simulink model "Helicopter_Model"  (R2025a)
settings: Solver=VariableStepAuto  StartTime=0.0  StopTime=10.0  RelTol=1e-3
settings Model: Creator=Admin  LastModifiedBy=Admin

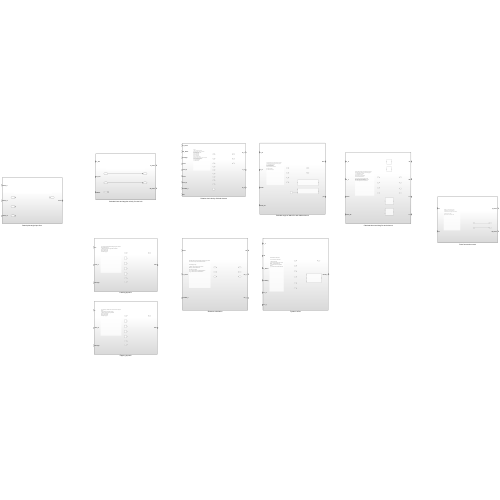
[thumbnail: Simulink's stored preview of the top-level diagram]
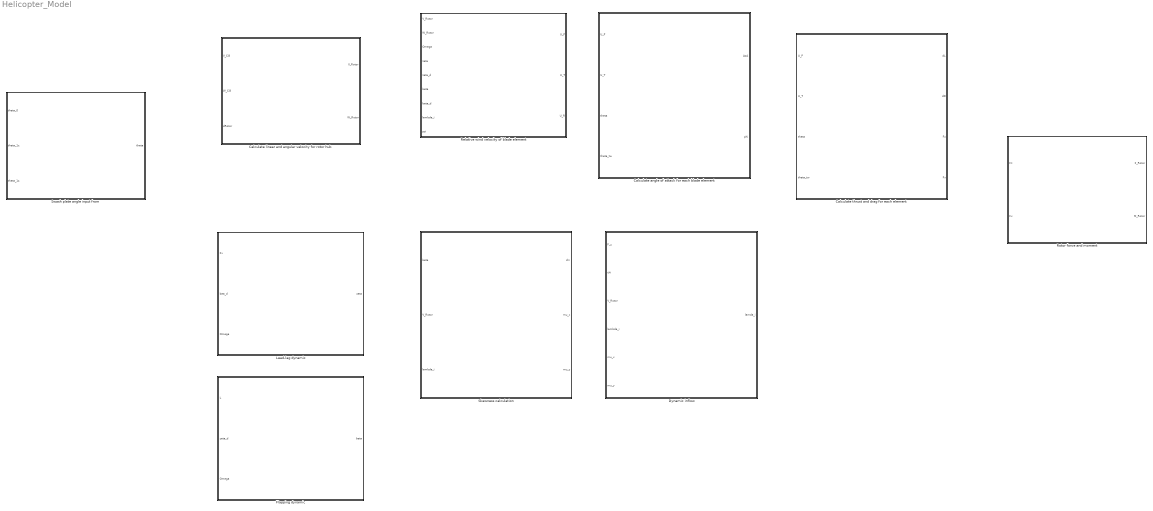
== system Helicopter_Model ==
  Calculate angle of attack for each blade element : Subsystem
  Calculate linear and angular velocity for rotor hub : Subsystem
  Calculate thrust and drag for each element : Subsystem
  Dynamic inflow : Subsystem
  Flapping dynamic : Subsystem
  Lead-lag dynamic : Subsystem
  Relative wind velocity of blade element : Subsystem
  Rotor force and moment : Subsystem
  Skewness calculation : Subsystem
  Swash plate angle input from : Subsystem

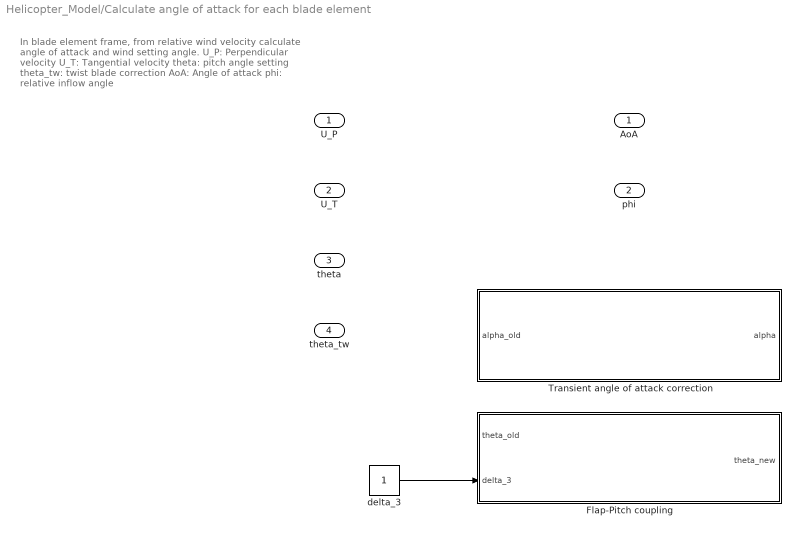
== system Helicopter_Model/Calculate angle of attack for each blade element ==
  note: In blade element frame, from relative wind velocity calculate angle of attack and wind setting angle.
      | U_P: Perpendicular velocity
      | U_T: Tangential velocity
      | theta: pitch angle setting
      | theta_tw: twist blade correction
      |
      | AoA: Angle of attack
      | phi: relative inflow angle
  U_P : Inport
  U_T : Inport  Port=2
  theta : Inport  Port=3
  theta_tw : Inport  Port=4
  Flap-Pitch coupling : Subsystem
  Transient angle of attack correction : Subsystem
  delta_3 : Constant
  AoA : Outport
  phi : Outport  Port=2
  wires:
  delta_3/1 -> Flap-Pitch coupling/2(delta_3)

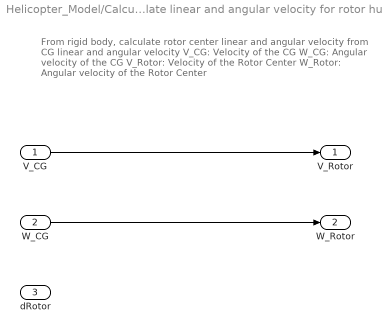
== system Helicopter_Model/Calculate linear and angular velocity for rotor hub ==
  note: From rigid body, calculate rotor center linear and angular velocity
      |  from CG linear and angular velocity
      | V_CG: Velocity of the CG
      | W_CG: Angular velocity of the CG
      | V_Rotor: Velocity of the Rotor Center
      | W_Rotor: Angular velocity of the Rotor Center
  V_CG : Inport
  W_CG : Inport  Port=2
  dRotor : Inport  Port=3
  V_Rotor : Outport
  W_Rotor : Outport  Port=2
  wires:
  V_CG/1 -> V_Rotor/1
  W_CG/1 -> W_Rotor/1

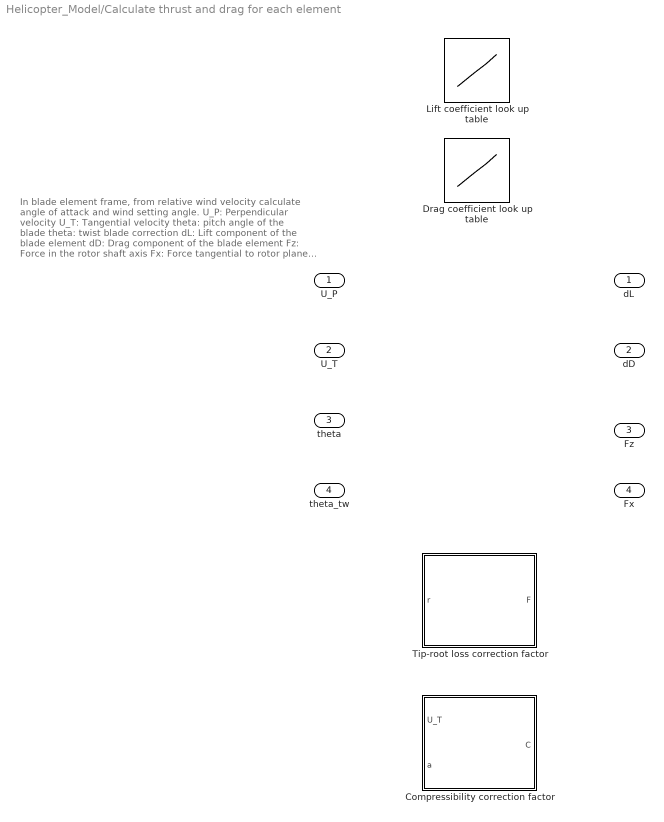
== system Helicopter_Model/Calculate thrust and drag for each element ==
  note: In blade element frame, from relative wind velocity calculate angle of attack and wind setting angle.
      | U_P: Perpendicular velocity
      | U_T: Tangential velocity
      | theta: pitch angle of the blade
      | theta: twist blade correction
      |
      | dL: Lift component of the blade element
      | dD: Drag component of the blade element
      | Fz: Force in the rotor shaft axis
      | Fx: Force tangential to rotor plane axis
  U_P : Inport
  U_T : Inport  Port=2
  theta : Inport  Port=3
  theta_tw : Inport  Port=4
  Compressibility correction factor : Subsystem
  Drag coefficient look up table : Lookup_n-D  NumberOfTableDimensions=1  BreakpointsForDimension1=[-5:5]  Table=tanh([-5:5])  InternalRulePriority=Speed  RndMeth=Simplest
  Lift coefficient look up table : Lookup_n-D  NumberOfTableDimensions=1  BreakpointsForDimension1=[-5:5]  Table=tanh([-5:5])  InternalRulePriority=Speed  RndMeth=Simplest
  Tip-root loss correction factor : Subsystem
  dL : Outport
  dD : Outport  Port=2
  Fz : Outport  Port=3
  Fx : Outport  Port=4

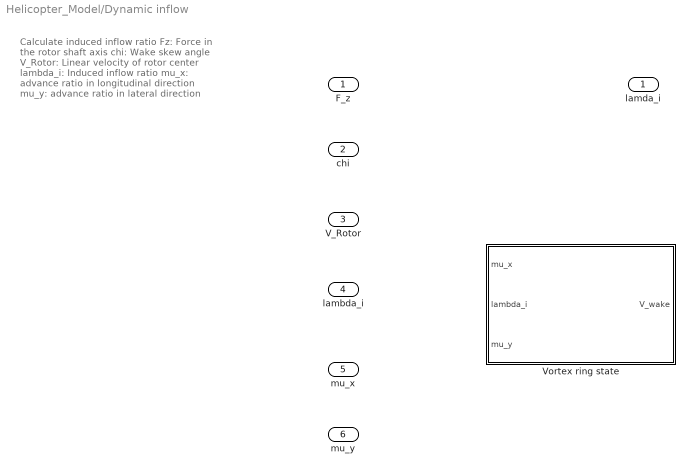
== system Helicopter_Model/Dynamic inflow ==
  note: Calculate induced inflow ratio
      |
      | Fz: Force in the rotor shaft axis
      |
      | chi: Wake skew angle
      | V_Rotor: Linear velocity of rotor center
      | lambda_i: Induced inflow ratio
      | mu_x: advance ratio in longitudinal direction
      | mu_y: advance ratio in lateral direction
  F_z : Inport
  chi : Inport  Port=2
  V_Rotor : Inport  Port=3
  lambda_i : Inport  Port=4
  mu_x : Inport  Port=5
  mu_y : Inport  Port=6
  Vortex ring state : Subsystem
  lamda_i : Outport

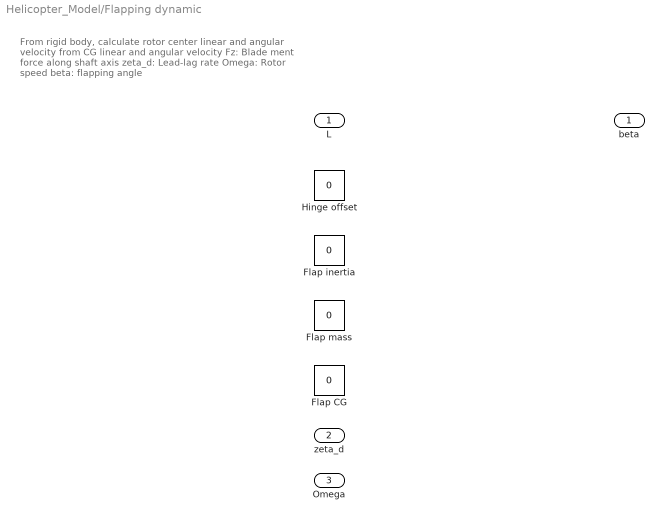
== system Helicopter_Model/Flapping dynamic ==
  note: From rigid body, calculate rotor center linear and angular velocity
      | from CG linear and angular velocity
      | Fz: Blade ment force along shaft axis
      | zeta_d: Lead-lag rate
      | Omega: Rotor speed
      | beta: flapping angle
  L : Inport
  zeta_d : Inport  Port=2
  Omega : Inport  Port=3
  Flap CG : Constant  Value=0
  Flap inertia : Constant  Value=0
  Flap mass : Constant  Value=0
  Hinge offset : Constant  Value=0
  beta : Outport

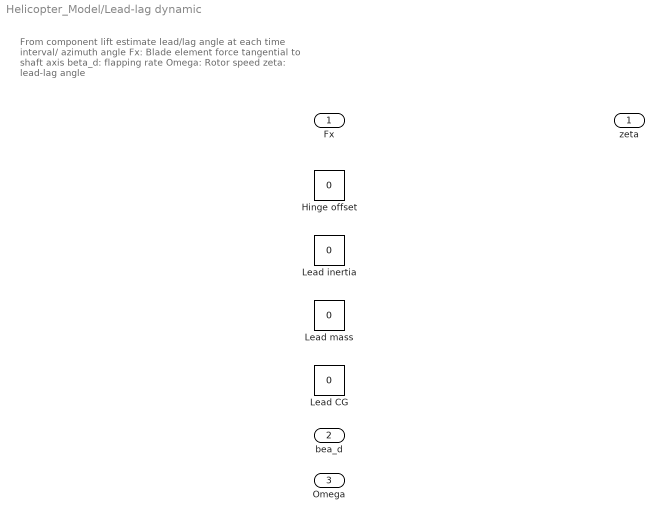
== system Helicopter_Model/Lead-lag dynamic ==
  note: From component lift estimate lead/lag angle at each time interval/ azimuth angle
      | Fx: Blade element force tangential to shaft axis
      | beta_d: flapping rate
      | Omega: Rotor speed
      | zeta: lead-lag angle
  Fx : Inport
  bea_d : Inport  Port=2
  Omega : Inport  Port=3
  Hinge offset : Constant  Value=0
  Lead CG : Constant  Value=0
  Lead inertia : Constant  Value=0
  Lead mass : Constant  Value=0
  zeta : Outport

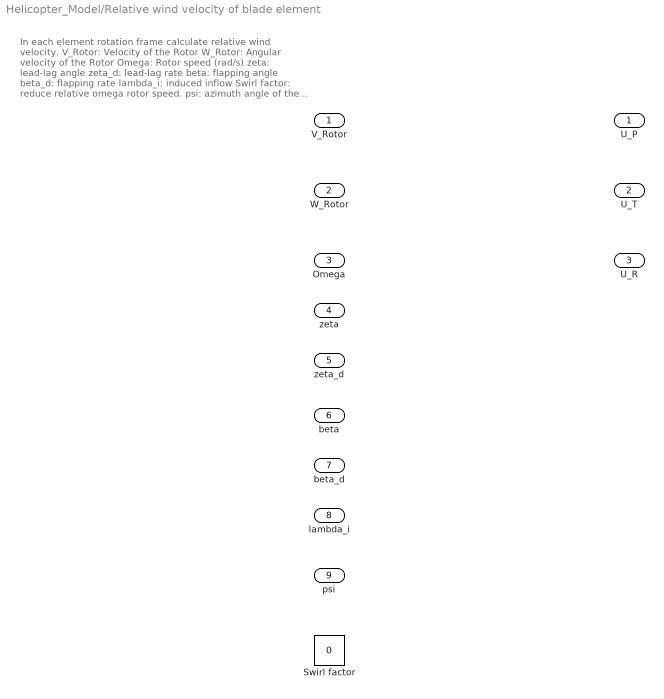
== system Helicopter_Model/Relative wind velocity of blade element ==
  note: In each element rotation frame calculate relative wind velocity.
      | V_Rotor: Velocity of the Rotor
      | W_Rotor: Angular velocity of the Rotor
      | Omega: Rotor speed (rad/s)
      | zeta: lead-lag angle
      | zeta_d: lead-lag rate
      | beta: flapping angle
      | beta_d: flapping rate
      | lambda_i: induced inflow
      | Swirl factor: reduce relative omega rotor speed.
      | psi: azimuth angle of the blade
      | U_P: Perpendicular velocity
      | U_T: Tangential velocity
      | U_R: Radial velocity
  V_Rotor : Inport
  W_Rotor : Inport  Port=2
  Omega : Inport  Port=3
  zeta : Inport  Port=4
  zeta_d : Inport  Port=5
  beta : Inport  Port=6
  beta_d : Inport  Port=7
  lambda_i : Inport  Port=8
  psi : Inport  Port=9
  Swirl factor : Constant  Value=0
  U_P : Outport
  U_T : Outport  Port=2
  U_R : Outport  Port=3

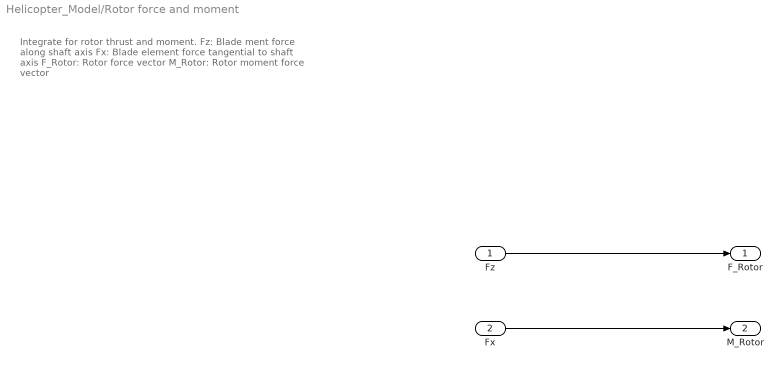
== system Helicopter_Model/Rotor force and moment ==
  note: Integrate for rotor thrust and moment.
      |
      | Fz: Blade ment force along shaft axis
      | Fx: Blade element force tangential to shaft axis
      |
      | F_Rotor: Rotor force vector
      | M_Rotor: Rotor moment force vector
  Fz : Inport
  Fx : Inport  Port=2
  F_Rotor : Outport
  M_Rotor : Outport  Port=2
  wires:
  Fz/1 -> F_Rotor/1
  Fx/1 -> M_Rotor/1

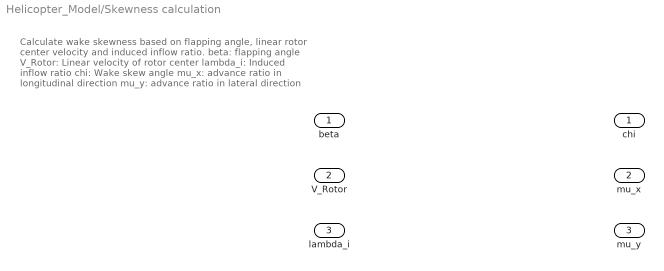
== system Helicopter_Model/Skewness calculation ==
  note: Calculate wake skewness based on flapping angle, linear rotor center velocity and induced inflow ratio.
      |
      | beta: flapping angle
      | V_Rotor: Linear velocity of rotor center
      | lambda_i: Induced inflow ratio
      |
      | chi: Wake skew angle
      | mu_x: advance ratio in longitudinal direction
      | mu_y: advance ratio in lateral direction
  beta : Inport
  V_Rotor : Inport  Port=2
  lambda_i : Inport  Port=3
  chi : Outport
  mu_x : Outport  Port=2
  mu_y : Outport  Port=3

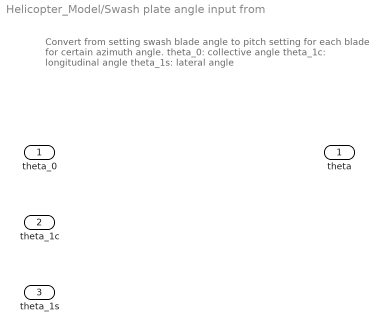
== system Helicopter_Model/Swash plate angle input from ==
  note: Convert from setting swash blade angle to pitch setting for each blade for certain azimuth angle.
      | theta_0: collective angle
      | theta_1c: longitudinal angle
      | theta_1s: lateral angle
  theta_0 : Inport
  theta_1c : Inport  Port=2
  theta_1s : Inport  Port=3
  theta : Outport

== system Helicopter_Model/Calculate angle of attack for each blade element/Flap-Pitch coupling ==
  note: Increase flap reduce pitch to compensate for lift
      | theta_old: pitch angle before flap coupling
      | delta_old: coupling factor
      | theta_new: pitch angle after flap coupling
  theta_old : Inport
  delta_3 : Inport  Port=2
  theta_new : Outport

== system Helicopter_Model/Calculate angle of attack for each blade element/Transient angle of attack correction ==
  note: Delay transient from angle of attack setting (Wagner)
      | alpha_old: intended angle of attack
      | alpha_new: current angle of attack status
  alpha_old : Inport
  alpha : Outport

== system Helicopter_Model/Calculate thrust and drag for each element/Compressibility correction factor ==
  note: Compressibility correction factor due to high Mach number
      |
      | U_T: Tangential velocity of the blade element
      | a: sound speed
      | C: Compresibility correction factor
  U_T : Inport
  a : Inport  Port=2
  C : Outport

== system Helicopter_Model/Calculate thrust and drag for each element/Tip-root loss correction factor ==
  note: Use Prandtl root-tip loss correction factor
      |
      | r: Normalized radius
      | F: Correction gain
  r : Inport
  F : Outport
  wires:
  r/1 -> F/1

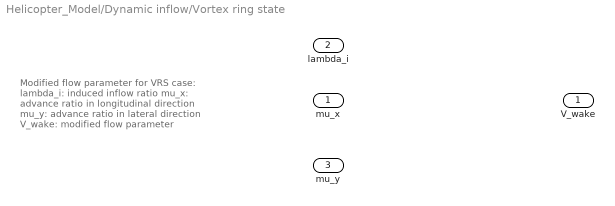
== system Helicopter_Model/Dynamic inflow/Vortex ring state ==
  note: Modified flow parameter for VRS case:
      | lambda_i: induced inflow ratio
      | mu_x: advance ratio in longitudinal direction
      | mu_y: advance ratio in lateral direction
      | V_wake: modified flow parameter
  mu_x : Inport
  lambda_i : Inport  Port=2
  mu_y : Inport  Port=3
  V_wake : Outport
